simulink model "myproject_exec"  (Simulink 3.00)
libraries: execlib x5

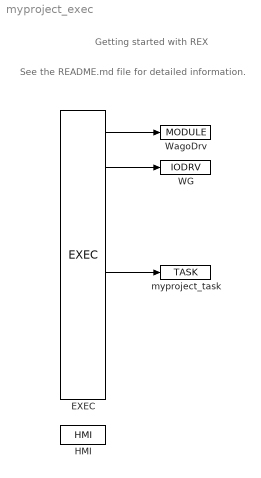
== system myproject_exec ==
  note: Getting started with REX
  note: See the README.md file for
      | detailed information.
  EXEC : execlib/EXEC  target=Generic target device  tick=0.02  ntick0=5  ntick1=50  ntick2=100  ntick3=1200  pri0=5  pri1=9  pri2=13  pri3=18
  HMI : execlib/HMI  IncludeHMI=on  HmiDir=hmi  SourceDir=hmisrc  GenerateWebWatch=off  GenerateRexHMI=on  RedirectToHMI=on  Compression=off
  WG : execlib/IODRV  module=WagoDrv  classname=WagoDrv  factor=1  stack=10240  pri=3  timer=off
  WagoDrv : execlib/MODULE
  myproject_task : execlib/TASK  factor=1  start=0  stop=1  stack=10240  MDLOPEN=on
  wires:
  EXEC/1 -> WagoDrv/1
  EXEC/2 -> WG/1
  EXEC/5 -> myproject_task/1
